simulink model "sistema_electromecanico"  (R2016b)
settings: Solver=VariableStepAuto  StartTime=0.0  StopTime=10.0  RelTol=1e-3
values from neighbouring files (symbols this model uses):
  Beq = bm+(bl)/r^2    (= 1.5e-05)    [c4ModeloCompleto_var.m]
  Cts = .818    (= 0.818)    [c4ModeloCompleto.m]    (also in c4ModeloCompleto_var.m)
  Jeq = Jm+(Jl/r^2)    (= 5.65099476805e-06)    [c4ModeloCompleto_var.m]
  Ld = 6.6    [c4ModeloCompleto.m]    (also in c4ModeloCompleto_var.m = 0.0066)
  Lq = 5.8    [c4ModeloCompleto.m]    (also in c4ModeloCompleto_var.m = 0.0058)
  Pp = 3    [c4ModeloCompleto.m]    (also in c4ModeloCompleto_var.m)
  r = 314.3008    [c4ModeloCompleto.m]    (also in c4ModeloCompleto_var.m)
  Rs = 1.02    [c4ModeloCompleto_var.m]
  Rts_amb = 146.7    [c4ModeloCompleto.m]    (also in c4ModeloCompleto_var.m)
undefined symbols (not defined in the file or in its folder): L0
settings Model: Creator=agustin  LastModifiedBy=agustin

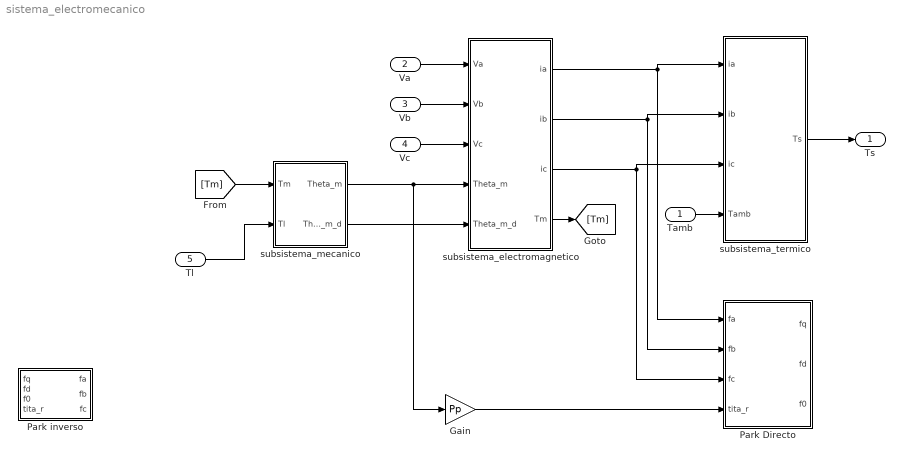
== system sistema_electromecanico ==
  Tamb : Inport
  Va : Inport  Port=2
  Vb : Inport  Port=3
  Vc : Inport  Port=4
  Tl : Inport  Port=5
  Gain : Gain  Gain=Pp
  Park Directo : MATLAB Function  TreatAsAtomicUnit=on
  Park inverso : MATLAB Function  TreatAsAtomicUnit=on
  "subsistema_electromagnetico " : Subsystem
  "subsistema_mecanico " : Subsystem
  subsistema_termico : Subsystem
  Ts : Outport
  wires:
  "subsistema_mecanico "/2("Theta_m_d ") -> "subsistema_electromagnetico "/5(Theta_m_d)
  subsistema_termico/1(Ts) -> Ts/1
  Tamb/1 -> subsistema_termico/4(Tamb)
  "subsistema_mecanico "/1("Theta_m ") -> Gain/1, "subsistema_electromagnetico "/4(Theta_m)
  Va/1 -> "subsistema_electromagnetico "/1(Va)
  Vb/1 -> "subsistema_electromagnetico "/2(Vb)
  Vc/1 -> "subsistema_electromagnetico "/3(Vc)
  "subsistema_electromagnetico "/1(ia) -> subsistema_termico/1(ia), Park Directo/1(fa)
  "subsistema_electromagnetico "/2(ib) -> subsistema_termico/2(ib), Park Directo/2(fb)
  "subsistema_electromagnetico "/3(ic) -> subsistema_termico/3("ic "), Park Directo/3(fc)
  Gain/1 -> Park Directo/4(tita_r)
  [Tm] -> "subsistema_mecanico "/1(Tm)
  "subsistema_electromagnetico "/4(Tm) -> [Tm]
  Tl/1 -> "subsistema_mecanico "/2(Tl)

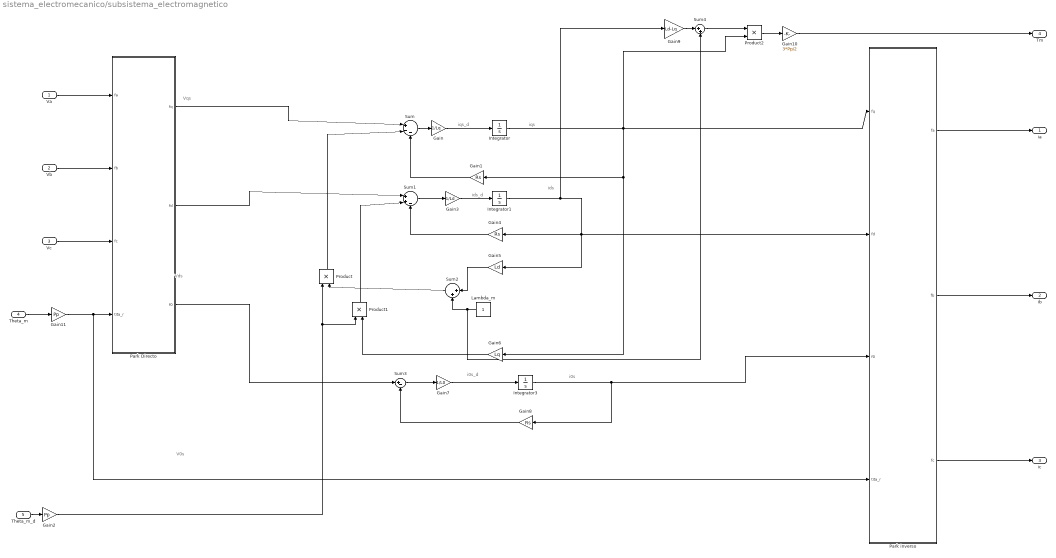
== system sistema_electromecanico/subsistema_electromagnetico  ==
  note: V0s
  note: Vds
  note: Vqs
  note: i0s
  note: i0s_d
  note: ids_d
  note: ids
  note: iqs
  note: iqs_d
  Va : Inport
  Vb : Inport  Port=2
  Vc : Inport  Port=3
  Theta_m : Inport  Port=4
  Theta_m_d : Inport  Port=5
  Gain : Gain  Gain=1/Lq
  Gain1 : Gain  Gain=Rs
  Gain10 : Gain  Gain=3*Pp/2
  Gain11 : Gain  Gain=Pp
  Gain2 : Gain  Gain=Pp
  Gain3 : Gain  Gain=1/Ld
  Gain4 : Gain  Gain=Rs
  Gain5 : Gain  Gain=Ld
  Gain6 : Gain  Gain=Lq
  Gain7 : Gain  Gain=1/L0
  Gain8 : Gain  Gain=Rs
  Gain9 : Gain  Gain=Ld-Lq
  Integrator : Integrator
  Integrator1 : Integrator
  Integrator3 : Integrator
  "Lambda_m " : Constant
  Park Directo : MATLAB Function  TreatAsAtomicUnit=on
  Park inverso : MATLAB Function  TreatAsAtomicUnit=on
  Product : Product
  Product1 : Product
  Product2 : Product
  Sum : Sum  Inputs=|+--
  Sum1 : Sum  Inputs=|++-
  Sum2 : Sum  Inputs=|++
  Sum3 : Sum  Inputs=|+-
  Sum4 : Sum  Inputs=|++
  ia : Outport
  ib : Outport  Port=2
  ic : Outport  Port=3
  Tm : Outport  Port=4
  wires:
  Product/1 -> Sum/2
  Theta_m_d/1 -> Gain2/1
  Product1/1 -> Sum1/2
  Gain2/1 -> Product1/1, Product/1
  Park Directo/3(f0) -> Sum3/1
  Integrator/1 -> Product2/2, Park inverso/1(fq), Gain1/1, Gain6/1
  Gain8/1 -> Sum3/2
  Sum2/1 -> Product/2
  Sum3/1 -> Gain7/1
  Park Directo/1(fq) -> Sum/1
  Sum/1 -> Gain/1
  Gain3/1 -> Integrator1/1
  Park Directo/2(fd) -> Sum1/1
  Gain4/1 -> Sum1/3
  Integrator1/1 -> Gain9/1, Gain5/1, Gain4/1, Park inverso/2(fd)
  Sum1/1 -> Gain3/1
  Gain5/1 -> Sum2/1
  Gain/1 -> Integrator/1
  Gain6/1 -> Product1/2
  Gain1/1 -> Sum/3
  "Lambda_m "/1 -> Sum4/2, Sum2/2
  Gain7/1 -> Integrator3/1
  Integrator3/1 -> Park inverso/3(f0), Gain8/1
  Gain9/1 -> Sum4/1
  Sum4/1 -> Product2/1
  Product2/1 -> Gain10/1
  Gain10/1 -> Tm/1
  Vb/1 -> Park Directo/2(fb)
  Va/1 -> Park Directo/1(fa)
  Vc/1 -> Park Directo/3(fc)
  Theta_m/1 -> Gain11/1
  Gain11/1 -> Park inverso/4(tita_r), Park Directo/4(tita_r)
  Park inverso/1(fa) -> ia/1
  Park inverso/2(fb) -> ib/1
  Park inverso/3(fc) -> ic/1

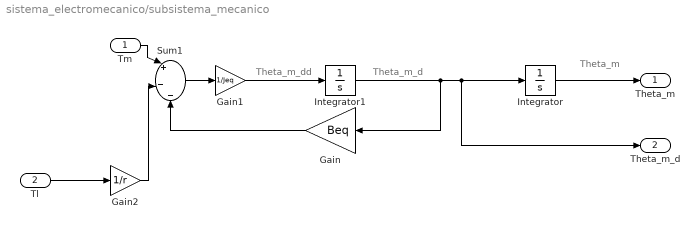
== system sistema_electromecanico/subsistema_mecanico  ==
  note: Theta_m_dd
  note: Theta_m_d
  note: Theta_m
  Tm : Inport
  Tl : Inport  Port=2
  Gain : Gain  Gain=Beq
  Gain1 : Gain  Gain=1/Jeq
  Gain2 : Gain  Gain=1/r
  Integrator : Integrator
  Integrator1 : Integrator
  Sum1 : Sum  Inputs=|+|-|-
  "Theta_m " : Outport
  "Theta_m_d " : Outport  Port=2
  wires:
  Gain1/1 -> Integrator1/1
  Integrator1/1 -> Gain/1, "Theta_m_d "/1, Integrator/1
  Integrator/1 -> "Theta_m "/1
  Sum1/1 -> Gain1/1
  Tm/1 -> Sum1/1
  Gain/1 -> Sum1/3
  Tl/1 -> Gain2/1
  Gain2/1 -> Sum1/2

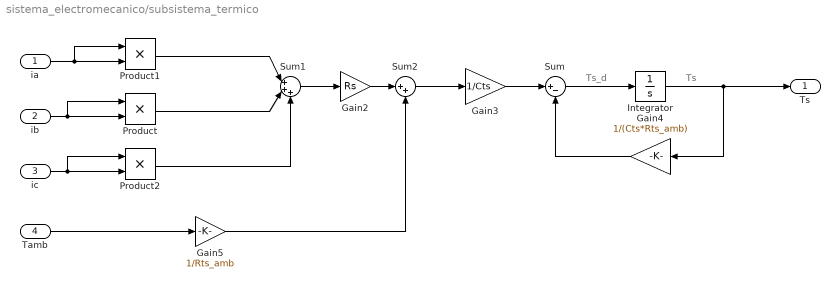
== system sistema_electromecanico/subsistema_termico ==
  note: Ts
  note: Ts_d
  ia : Inport
  ib : Inport  Port=2
  "ic " : Inport  Port=3
  Tamb : Inport  Port=4
  Gain2 : Gain  Gain=Rs
  Gain3 : Gain  Gain=1/Cts
  Gain4 : Gain  Gain=1/(Cts*Rts_amb)
  Gain5 : Gain  Gain=1/Rts_amb
  Integrator : Integrator
  Product : Product
  Product1 : Product
  Product2 : Product
  Sum : Sum  Inputs=|+-
  Sum1 : Sum  Inputs=|+++
  Sum2 : Sum  Inputs=|++
  Ts : Outport
  wires:
  Gain4/1 -> Sum/2
  Sum1/1 -> Gain2/1
  Product2/1 -> Sum1/3
  Product/1 -> Sum1/2
  Integrator/1 -> Gain4/1, Ts/1
  ib/1 -> Product/2, Product/1
  "ic "/1 -> Product2/2, Product2/1
  Sum/1 -> Integrator/1
  Gain3/1 -> Sum/1
  Sum2/1 -> Gain3/1
  Product1/1 -> Sum1/1
  Gain5/1 -> Sum2/2
  Gain2/1 -> Sum2/1
  ia/1 -> Product1/2, Product1/1
  Tamb/1 -> Gain5/1

== matlab function sistema_electromecanico/Park inverso ==
  data: fq input; fd input; f0 input; tita_r input; fa output; fb output; fc output
function [fa, fb, fc] = t_park_inv(fq, fd , f0, tita_r)


park_MATRIZ = [cos(tita_r)        sin(tita_r)        1; 
               cos(tita_r-2*pi/3) sin(tita_r-2*pi/3) 1;
               cos(tita_r+2*pi/3) sin(tita_r+2*pi/3) 1];
                 
park_inv = park_MATRIZ * [fq;fd;f0];
fa = park_inv(1);
fb = park_inv(2);
fc = park_inv(3);
end

== matlab function sistema_electromecanico/subsistema_electromagnetico /Park Directo ==
  data: fa input; fq output; fb input; fc input; tita_r input; fd output; f0 output
function [fq,fd,f0]     = t_park(fa,fb,fc,tita_r)

park_MATRIZ = [cos(tita_r) cos(tita_r-2*pi/3) cos(tita_r+2*pi/3); 
               sin(tita_r) sin(tita_r-2*pi/3) sin(tita_r+2*pi/3);
                  0.5           0.5            0.5];
                 
park_dir = (2/3) * park_MATRIZ * [fa;fb;fc];
fq = park_dir(1);
fd = park_dir(2);
f0 = park_dir(3);
end

== matlab function sistema_electromecanico/subsistema_electromagnetico /Park inverso ==
  data: fq input; fd input; f0 input; tita_r input; fa output; fb output; fc output
function [fa, fb, fc] = t_park_inv(fq, fd , f0, tita_r)


park_MATRIZ = [cos(tita_r)        sin(tita_r)        1; 
               cos(tita_r-2*pi/3) sin(tita_r-2*pi/3) 1;
               cos(tita_r+2*pi/3) sin(tita_r+2*pi/3) 1];
                 
park_inv = park_MATRIZ * [fq;fd;f0];
fa = park_inv(1);
fb = park_inv(2);
fc = park_inv(3);
end

== matlab function sistema_electromecanico/Park Directo ==
  data: fa input; fq output; fb input; fc input; tita_r input; fd output; f0 output
function [fq,fd,f0]     = t_park(fa,fb,fc,tita_r)

park_MATRIZ = [cos(tita_r) cos(tita_r-2*pi/3) cos(tita_r+2*pi/3); 
               sin(tita_r) sin(tita_r-2*pi/3) sin(tita_r+2*pi/3);
                  0.5           0.5            0.5];
                 
park_dir = (2/3) * park_MATRIZ * [fa;fb;fc];
fq = park_dir(1);
fd = park_dir(2);
f0 = park_dir(3);
end
